simulink library "HexapodLib"  (R2014b)
settings: Solver=ode45  StartTime=0.0  StopTime=10.0  RelTol=1e-3
undefined symbols (not defined in the file): X, Y, Z
libraries: nesl_utility x95, sm_lib x85, HexapodLib x15, Contact_Forces_Lib x12
(part 2 of 3)

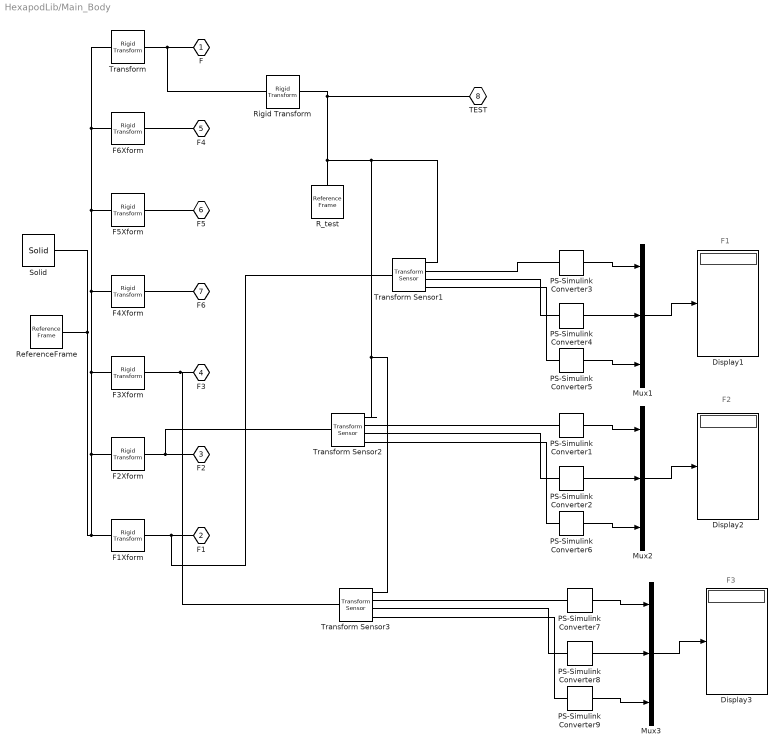
== system HexapodLib/Main_Body ==
  note: F1
  note: F2
  note: F3
  Display1 : Display
  Display2 : Display
  Display3 : Display
  F1Xform : sm_lib/Frames and Transforms/Rigid Transform  TranslationMethod=Cartesian  TranslationLengthUnit=mm  TranslationStandardAxis=+Z  TranslationStandardOffset=0  TranslationCartesianOffset=[60.910077554195617 -121.91007755419609 -2.5999999999923125]  TranslationROffset=0  TranslationROffsetUnits=m  TranslationZOffset=0  TranslationZOffsetUnits=m  TranslationThetaOffset=0  TranslationThetaOffsetUnits=deg  RotationMethod=ArbitraryAxis  RotationAngleUnits=rad  RotationStandardAxis=+Z  RotationAngle=2.3561944901923448  RotationArbitraryAxis=[-5.0947287514427085e-14 -3.4119027764489725e-14 -1]  FollAlignAxisA=+X  BaseAlignAxisA=+Y  FollAlignAxisB=+Y  BaseAlignAxisB=+Z  RotationMatrix=[1 0 0; 0 1 0; 0 0 1]  BlockFunction=simmechanics.library.frames_transforms.rigid_transform
  F2Xform : sm_lib/Frames and Transforms/Rigid Transform  TranslationMethod=Cartesian  TranslationLengthUnit=mm  TranslationStandardAxis=+Z  TranslationStandardOffset=0  TranslationCartesianOffset=[103.49999999999983 0 -2.6000000000064678]  TranslationROffset=0  TranslationROffsetUnits=m  TranslationZOffset=0  TranslationZOffsetUnits=m  TranslationThetaOffset=0  TranslationThetaOffsetUnits=deg  RotationMethod=ArbitraryAxis  RotationAngleUnits=rad  RotationStandardAxis=+Z  RotationAngle=1.5707963267948968  RotationArbitraryAxis=[-7.8558330123970482e-14 -1.5711666024794097e-14 -1]  FollAlignAxisA=+X  BaseAlignAxisA=+Y  FollAlignAxisB=+Y  BaseAlignAxisB=+Z  RotationMatrix=[1 0 0; 0 1 0; 0 0 1]  BlockFunction=simmechanics.library.frames_transforms.rigid_transform
  F3Xform : sm_lib/Frames and Transforms/Rigid Transform  TranslationMethod=Cartesian  TranslationLengthUnit=mm  TranslationStandardAxis=+Z  TranslationStandardOffset=0  TranslationCartesianOffset=[60.910077554195631 121.91007755419552 -2.6000000000152843]  TranslationROffset=0  TranslationROffsetUnits=m  TranslationZOffset=0  TranslationZOffsetUnits=m  TranslationThetaOffset=0  TranslationThetaOffsetUnits=deg  RotationMethod=ArbitraryAxis  RotationAngleUnits=rad  RotationStandardAxis=+Z  RotationAngle=0.7853981633974495  RotationArbitraryAxis=[-1.4521728366319145e-13 2.8727636334686562e-14 -1]  FollAlignAxisA=+X  BaseAlignAxisA=+Y  FollAlignAxisB=+Y  BaseAlignAxisB=+Z  RotationMatrix=[1 0 0; 0 1 0; 0 0 1]  BlockFunction=simmechanics.library.frames_transforms.rigid_transform
  F4Xform : sm_lib/Frames and Transforms/Rigid Transform  TranslationMethod=Cartesian  TranslationLengthUnit=mm  TranslationStandardAxis=+Z  TranslationStandardOffset=0  TranslationCartesianOffset=[-60.910077554195958 121.91007755419555 -2.6000000000076282]  TranslationROffset=0  TranslationROffsetUnits=m  TranslationZOffset=0  TranslationZOffsetUnits=m  TranslationThetaOffset=0  TranslationThetaOffsetUnits=deg  RotationMethod=ArbitraryAxis  RotationAngleUnits=rad  RotationStandardAxis=+Z  RotationAngle=0.78539816339744906  RotationArbitraryAxis=[-8.2370619564015128e-14 1.229976324834512e-13 1]  FollAlignAxisA=+X  BaseAlignAxisA=+Y  FollAlignAxisB=+Y  BaseAlignAxisB=+Z  RotationMatrix=[1 0 0; 0 1 0; 0 0 1]  BlockFunction=simmechanics.library.frames_transforms.rigid_transform
  F5Xform : sm_lib/Frames and Transforms/Rigid Transform  TranslationMethod=Cartesian  TranslationLengthUnit=mm  TranslationStandardAxis=+Z  TranslationStandardOffset=0  TranslationCartesianOffset=[-103.50000000000016 0 -2.5999999999934662]  TranslationROffset=0  TranslationROffsetUnits=m  TranslationZOffset=0  TranslationZOffsetUnits=m  TranslationThetaOffset=0  TranslationThetaOffsetUnits=deg  RotationMethod=ArbitraryAxis  RotationAngleUnits=rad  RotationStandardAxis=+Z  RotationAngle=1.5707963267948968  RotationArbitraryAxis=[-1.5711666024794097e-14 7.8558330123970482e-14 1]  FollAlignAxisA=+X  BaseAlignAxisA=+Y  FollAlignAxisB=+Y  BaseAlignAxisB=+Z  RotationMatrix=[1 0 0; 0 1 0; 0 0 1]  BlockFunction=simmechanics.library.frames_transforms.rigid_transform
  F6Xform : sm_lib/Frames and Transforms/Rigid Transform  TranslationMethod=Cartesian  TranslationLengthUnit=mm  TranslationStandardAxis=+Z  TranslationStandardOffset=0  TranslationCartesianOffset=[-60.910077554195937 -121.91007755419606 -2.5999999999846568]  TranslationROffset=0  TranslationROffsetUnits=m  TranslationZOffset=0  TranslationZOffsetUnits=m  TranslationThetaOffset=0  TranslationThetaOffsetUnits=deg  RotationMethod=ArbitraryAxis  RotationAngleUnits=rad  RotationStandardAxis=+Z  RotationAngle=2.3561944901923453  RotationArbitraryAxis=[1.1899376584749339e-14 6.0150968384274875e-14 1]  FollAlignAxisA=+X  BaseAlignAxisA=+Y  FollAlignAxisB=+Y  BaseAlignAxisB=+Z  RotationMatrix=[1 0 0; 0 1 0; 0 0 1]  BlockFunction=simmechanics.library.frames_transforms.rigid_transform
  Mux1 : Mux  Inputs=3
  Mux2 : Mux  Inputs=3
  Mux3 : Mux  Inputs=3
  PS-Simulink Converter{1..9} (9 alike) : nesl_utility/PS-Simulink Converter  PhysicalDomain=network_engine_domain  SubClassName=ps_output  LeftPortType=input  RightPortType=output  PseudoPeriodic=off  Frequencies=[]  Unit=mm  AffineConversion=off
  R_test : sm_lib/Frames and Transforms/Reference Frame  BlockFunction=simmechanics.library.frames_transforms.reference_frame
  ReferenceFrame : sm_lib/Frames and Transforms/Reference Frame  BlockFunction=simmechanics.library.frames_transforms.reference_frame
  Rigid Transform : sm_lib/Frames and Transforms/Rigid Transform  TranslationMethod=None  TranslationLengthUnit=m  TranslationStandardAxis=+Z  TranslationStandardOffset=0  TranslationCartesianOffset=[0 0 0]  TranslationROffset=0  TranslationROffsetUnits=m  TranslationZOffset=0  TranslationZOffsetUnits=m  TranslationThetaOffset=0  TranslationThetaOffsetUnits=deg  RotationMethod=StandardAxis  RotationAngleUnits=deg  RotationStandardAxis=+Z  RotationAngle=-180  RotationArbitraryAxis=[0 0 1]  FollAlignAxisA=+X  BaseAlignAxisA=+Y  FollAlignAxisB=+Y  BaseAlignAxisB=+Z  RotationMatrix=[1 0 0; 0 1 0; 0 0 1]  BlockFunction=simmechanics.library.frames_transforms.rigid_transform
  Solid : sm_lib/Body Elements/Solid  InertiaType=Custom  Mass=0.63100000000000001  MassUnits=kg  CenterOfMass=[2.0291292946603825 -3.6242909829433687 -16.352184508248953]  CenterOfMassUnits=mm  MomentsOfInertia=[273.36575860845227 90.65491799060328 363.95192659905558]  MomentsOfInertiaUnits=kg*mm^2  ProductsOfInertia=[0 0 0]  ProductsOfInertiaUnits=kg*mm^2  DensityBased=on  Density=1000  DensityUnits=kg/(m^3)  GraphicType=FromGeometry  MarkerShape=Sphere  MarkerSize=10  MarkerSizeUnits=m  GraphicVisPropType=SimpleVisualProperties  GraphicDiffuseColor=[0.50196078431372548 0.50196078431372548 0.50196078431372548]  GraphicSpecularColor=[0.5 0.5 0.5 1.0]  GraphicAmbientColor=[0.15 0.15 0.15 1.0]  GraphicEmissiveColor=[0.0 0.0 0.0 1.0]  GraphicShininess=75  GraphicOpacity=1  GeometryShape=FromFile  RectangleSize=[1 1]  RectangleSizeUnits=m  BrickDimensions=[1 1 1]  BrickDimensionUnits=m  CylinderRadius=1  CylinderRadiusUnits=m  CylinderLength=1  CylinderLengthUnits=m  SphereRadius=1  SphereRadiusUnits=m  EllipsoidRadii=[1 1 1]  EllipsoidRadiiUnits=m  ExtrusionCrossSection=[1 1; -1 1; -1 -1; 1 -1]  ExtrusionCrossSectionUnits=m  ExtrusionLength=1  ExtrusionLengthUnits=m  PolygonNumSides=3  PolygonOuterRadius=1  PolygonOuterRadiusUnits=m  ExtGeomFileType=STL  ExtGeomFileName=Main_body_Default_sldprt.STL  ExtGeomFileUnits=mm  RevolutionCrossSection=[1 1; 1 -1; 2 -1; 2 1]  RevolutionCrossSectionUnits=m  RevolutionExtent=Full  RevolutionAngle=180  RevolutionAngleUnits=deg  BlockFunction=simmechanics.library.body_elements.solid
  Transform : sm_lib/Frames and Transforms/Rigid Transform  TranslationMethod=Cartesian  TranslationLengthUnit=mm  TranslationStandardAxis=+Z  TranslationStandardOffset=0  TranslationCartesianOffset=[0 0 0]  TranslationROffset=0  TranslationROffsetUnits=m  TranslationZOffset=0  TranslationZOffsetUnits=m  TranslationThetaOffset=0  TranslationThetaOffsetUnits=deg  RotationMethod=ArbitraryAxis  RotationAngleUnits=rad  RotationStandardAxis=+Z  RotationAngle=0  RotationArbitraryAxis=[0 0 0]  FollAlignAxisA=+X  BaseAlignAxisA=+Y  FollAlignAxisB=+Y  BaseAlignAxisB=+Z  RotationMatrix=[1 0 0; 0 1 0; 0 0 1]  BlockFunction=simmechanics.library.frames_transforms.rigid_transform
  Transform Sensor1 : sm_lib/Frames and Transforms/Transform Sensor  MeasurementFrame=Base  SenseAngle=off  SenseAxis=off  SenseAngle1=off  SenseAngle2=off  SenseAngle3=off  SenseQ=off  SenseR=off  SenseOmegaX=off  SenseOmegaY=off  SenseOmegaZ=off  SenseOmega1=off  SenseOmega2=off  SenseOmega3=off  SenseQDot=off  SenseRDot=off  SenseAlphaX=off  SenseAlphaY=off  SenseAlphaZ=off  SenseAlpha1=off  SenseAlpha2=off  SenseAlpha3=off  SenseQDDot=off  SenseRDDot=off  SenseX=on  SenseY=on  SenseZ=on  SenseRad=off  SenseAzim=off  SenseDist=off  SenseInc=off  SenseXDot=off  SenseYDot=off  SenseZDot=off  SenseRadDot=off  SenseAzimDot=off  SenseDistDot=off  SenseIncDot=off  SenseXDDot=off  SenseYDDot=off  SenseZDDot=off  SenseRadDDot=off  SenseAzimDDot=off  SenseDistDDot=off  SenseIncDDot=off  BlockFunction=simmechanics.library.frames_transforms.transform_sensor
  Transform Sensor2 : sm_lib/Frames and Transforms/Transform Sensor  MeasurementFrame=Base  SenseAngle=off  SenseAxis=off  SenseAngle1=off  SenseAngle2=off  SenseAngle3=off  SenseQ=off  SenseR=off  SenseOmegaX=off  SenseOmegaY=off  SenseOmegaZ=off  SenseOmega1=off  SenseOmega2=off  SenseOmega3=off  SenseQDot=off  SenseRDot=off  SenseAlphaX=off  SenseAlphaY=off  SenseAlphaZ=off  SenseAlpha1=off  SenseAlpha2=off  SenseAlpha3=off  SenseQDDot=off  SenseRDDot=off  SenseX=on  SenseY=on  SenseZ=on  SenseRad=off  SenseAzim=off  SenseDist=off  SenseInc=off  SenseXDot=off  SenseYDot=off  SenseZDot=off  SenseRadDot=off  SenseAzimDot=off  SenseDistDot=off  SenseIncDot=off  SenseXDDot=off  SenseYDDot=off  SenseZDDot=off  SenseRadDDot=off  SenseAzimDDot=off  SenseDistDDot=off  SenseIncDDot=off  BlockFunction=simmechanics.library.frames_transforms.transform_sensor
  Transform Sensor3 : sm_lib/Frames and Transforms/Transform Sensor  MeasurementFrame=Base  SenseAngle=off  SenseAxis=off  SenseAngle1=off  SenseAngle2=off  SenseAngle3=off  SenseQ=off  SenseR=off  SenseOmegaX=off  SenseOmegaY=off  SenseOmegaZ=off  SenseOmega1=off  SenseOmega2=off  SenseOmega3=off  SenseQDot=off  SenseRDot=off  SenseAlphaX=off  SenseAlphaY=off  SenseAlphaZ=off  SenseAlpha1=off  SenseAlpha2=off  SenseAlpha3=off  SenseQDDot=off  SenseRDDot=off  SenseX=on  SenseY=on  SenseZ=on  SenseRad=off  SenseAzim=off  SenseDist=off  SenseInc=off  SenseXDot=off  SenseYDot=off  SenseZDot=off  SenseRadDot=off  SenseAzimDot=off  SenseDistDot=off  SenseIncDot=off  SenseXDDot=off  SenseYDDot=off  SenseZDDot=off  SenseRadDDot=off  SenseAzimDDot=off  SenseDistDDot=off  SenseIncDDot=off  BlockFunction=simmechanics.library.frames_transforms.transform_sensor
  F : PMIOPort  Port=1  Side=Left
  F1 : PMIOPort  Port=2  Side=Left
  F2 : PMIOPort  Port=3  Side=Left
  F3 : PMIOPort  Port=4  Side=Left
  F4 : PMIOPort  Port=5  Side=Right
  F5 : PMIOPort  Port=6  Side=Right
  F6 : PMIOPort  Port=7  Side=Right
  TEST : PMIOPort  Port=8  Side=Right
  wires:
  Mux1/1 -> Display1/1
  PS-Simulink Converter5/1 -> Mux1/3
  PS-Simulink Converter4/1 -> Mux1/2
  PS-Simulink Converter3/1 -> Mux1/1
  Mux2/1 -> Display2/1
  PS-Simulink Converter6/1 -> Mux2/3
  PS-Simulink Converter2/1 -> Mux2/2
  PS-Simulink Converter1/1 -> Mux2/1
  Mux3/1 -> Display3/1
  PS-Simulink Converter9/1 -> Mux3/3
  PS-Simulink Converter8/1 -> Mux3/2
  PS-Simulink Converter7/1 -> Mux3/1
  connections:
  F2Xform/LConn1 -- F6Xform/LConn1 -- Transform/LConn1 -- F5Xform/LConn1 -- F4Xform/LConn1 -- F3Xform/LConn1 -- F1Xform/LConn1 -- Solid/RConn1 -- ReferenceFrame/RConn1
  F1Xform/RConn1 -- Transform Sensor1/LConn1 -- F1/RConn1
  F2Xform/RConn1 -- Transform Sensor2/LConn1 -- F2/RConn1
  F3Xform/RConn1 -- Transform Sensor3/LConn1 -- F3/RConn1
  F4Xform/RConn1 -- F6/RConn1
  F5Xform/RConn1 -- F5/RConn1
  F6Xform/RConn1 -- F4/RConn1
  Transform/RConn1 -- Rigid Transform/LConn1 -- F/RConn1
  R_test/RConn1 -- Transform Sensor2/RConn1 -- Transform Sensor3/RConn1 -- Transform Sensor1/RConn1 -- TEST/RConn1 -- Rigid Transform/RConn1
  Transform Sensor1/RConn4 -- PS-Simulink Converter5/LConn1
  PS-Simulink Converter3/LConn1 -- Transform Sensor1/RConn2
  PS-Simulink Converter4/LConn1 -- Transform Sensor1/RConn3
  PS-Simulink Converter1/LConn1 -- Transform Sensor2/RConn2
  PS-Simulink Converter2/LConn1 -- Transform Sensor2/RConn3
  Transform Sensor2/RConn4 -- PS-Simulink Converter6/LConn1
  PS-Simulink Converter8/LConn1 -- Transform Sensor3/RConn3
  PS-Simulink Converter7/LConn1 -- Transform Sensor3/RConn2
  Transform Sensor3/RConn4 -- PS-Simulink Converter9/LConn1

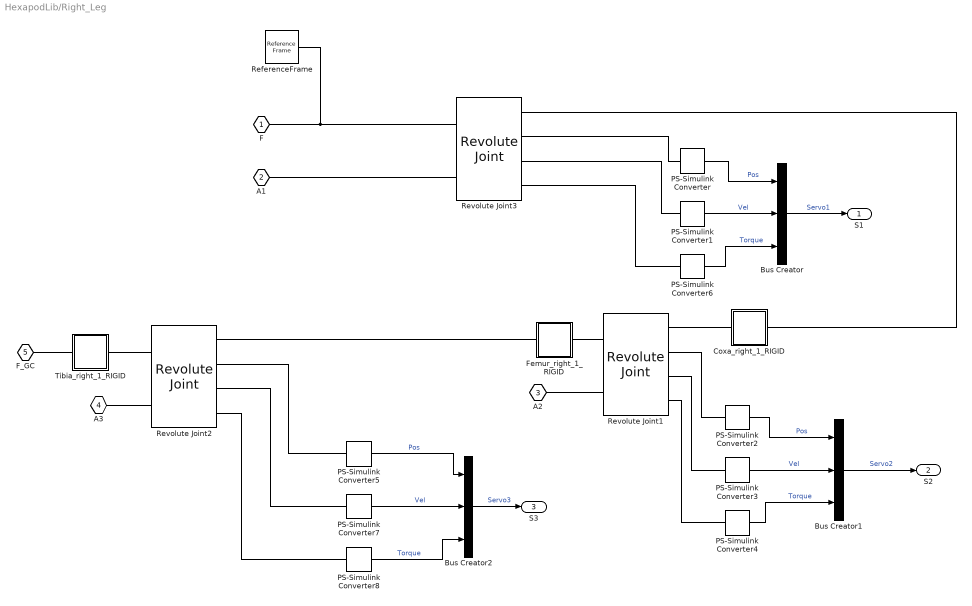
== system HexapodLib/Right_Leg ==
  Bus Creator : BusCreator  Inputs=3  OutDataTypeStr=Bus: Mes_servo
      settings: InheritFromInputs=off
  Bus Creator1 : BusCreator  Inputs=3  OutDataTypeStr=Bus: Mes_servo
      settings: InheritFromInputs=off
  Bus Creator2 : BusCreator  Inputs=3  OutDataTypeStr=Bus: Mes_servo
      settings: InheritFromInputs=off
  Coxa_right_1_RIGID : Subsystem
  Femur_right_1_RIGID : Subsystem
  PS-Simulink Converter : nesl_utility/PS-Simulink Converter  PhysicalDomain=network_engine_domain  SubClassName=ps_output  LeftPortType=input  RightPortType=output  PseudoPeriodic=off  Frequencies=[]  Unit=rad  AffineConversion=off
  PS-Simulink Converter1 : nesl_utility/PS-Simulink Converter  PhysicalDomain=network_engine_domain  SubClassName=ps_output  LeftPortType=input  RightPortType=output  PseudoPeriodic=off  Frequencies=[]  Unit=rad/s  AffineConversion=off
  PS-Simulink Converter2 : nesl_utility/PS-Simulink Converter  PhysicalDomain=network_engine_domain  SubClassName=ps_output  LeftPortType=input  RightPortType=output  PseudoPeriodic=off  Frequencies=[]  Unit=rad  AffineConversion=off
  PS-Simulink Converter3 : nesl_utility/PS-Simulink Converter  PhysicalDomain=network_engine_domain  SubClassName=ps_output  LeftPortType=input  RightPortType=output  PseudoPeriodic=off  Frequencies=[]  Unit=rad/s  AffineConversion=off
  PS-Simulink Converter4 : nesl_utility/PS-Simulink Converter  PhysicalDomain=network_engine_domain  SubClassName=ps_output  LeftPortType=input  RightPortType=output  PseudoPeriodic=off  Frequencies=[]  Unit=N*m  AffineConversion=off
  PS-Simulink Converter5 : nesl_utility/PS-Simulink Converter  PhysicalDomain=network_engine_domain  SubClassName=ps_output  LeftPortType=input  RightPortType=output  PseudoPeriodic=off  Frequencies=[]  Unit=rad  AffineConversion=off
  PS-Simulink Converter6 : nesl_utility/PS-Simulink Converter  PhysicalDomain=network_engine_domain  SubClassName=ps_output  LeftPortType=input  RightPortType=output  PseudoPeriodic=off  Frequencies=[]  Unit=N*m  AffineConversion=off
  PS-Simulink Converter7 : nesl_utility/PS-Simulink Converter  PhysicalDomain=network_engine_domain  SubClassName=ps_output  LeftPortType=input  RightPortType=output  PseudoPeriodic=off  Frequencies=[]  Unit=rad/s  AffineConversion=off
  PS-Simulink Converter8 : nesl_utility/PS-Simulink Converter  PhysicalDomain=network_engine_domain  SubClassName=ps_output  LeftPortType=input  RightPortType=output  PseudoPeriodic=off  Frequencies=[]  Unit=N*m  AffineConversion=off
  ReferenceFrame : sm_lib/Frames and Transforms/Reference Frame  BlockFunction=simmechanics.library.frames_transforms.reference_frame
  Revolute Joint1 : sm_lib/Joints/Revolute Joint  SenseConstraintForce=off  SenseConstraintForceX=off  SenseConstraintForceY=off  SenseConstraintForceZ=off  SenseConstraintTorque=off  SenseConstraintTorqueX=off  SenseConstraintTorqueY=off  SenseConstraintTorqueZ=off  SenseTotalForce=off  SenseTotalForceX=off  SenseTotalForceY=off  SenseTotalForceZ=off  SenseTotalTorque=off  SenseTotalTorqueX=off  SenseTotalTorqueY=off  SenseTotalTorqueZ=off  CompositeWrenchDir=FollowerOnBase  CompositeWrenchFrame=BaseFrame  EquilibriumPosition=0  EquilibriumPositionUnits=deg  SpringStiffness=spring_stiff  SpringStiffnessUnits=N*m/deg  DampingCoefficient=damping_coeff  DampingCoefficientUnits=N*m/(deg/s)  TorqueActuationMode=ComputedTorque  MotionActuationMode=InputMotion  SensePosition=on  SenseVelocity=on  SenseAcceleration=off  SenseTorqueForce=on  PositionTargetValue=0  PositionTargetValueUnits=deg  PositionTargetSpecify=off  PositionTargetPriority=High  VelocityTargetValue=0  VelocityTargetValueUnits=deg/s  VelocityTargetSpecify=off  VelocityTargetPriority=High  BlockFunction=simmechanics.library.joints.revolute_joint
  Revolute Joint2 : sm_lib/Joints/Revolute Joint  SenseConstraintForce=off  SenseConstraintForceX=off  SenseConstraintForceY=off  SenseConstraintForceZ=off  SenseConstraintTorque=off  SenseConstraintTorqueX=off  SenseConstraintTorqueY=off  SenseConstraintTorqueZ=off  SenseTotalForce=off  SenseTotalForceX=off  SenseTotalForceY=off  SenseTotalForceZ=off  SenseTotalTorque=off  SenseTotalTorqueX=off  SenseTotalTorqueY=off  SenseTotalTorqueZ=off  CompositeWrenchDir=FollowerOnBase  CompositeWrenchFrame=BaseFrame  EquilibriumPosition=0  EquilibriumPositionUnits=deg  SpringStiffness=spring_stiff  SpringStiffnessUnits=N*m/deg  DampingCoefficient=damping_coeff  DampingCoefficientUnits=N*m/(deg/s)  TorqueActuationMode=ComputedTorque  MotionActuationMode=InputMotion  SensePosition=on  SenseVelocity=on  SenseAcceleration=off  SenseTorqueForce=on  PositionTargetValue=0  PositionTargetValueUnits=deg  PositionTargetSpecify=off  PositionTargetPriority=High  VelocityTargetValue=0  VelocityTargetValueUnits=deg/s  VelocityTargetSpecify=off  VelocityTargetPriority=High  BlockFunction=simmechanics.library.joints.revolute_joint
  Revolute Joint3 : sm_lib/Joints/Revolute Joint  SenseConstraintForce=off  SenseConstraintForceX=off  SenseConstraintForceY=off  SenseConstraintForceZ=off  SenseConstraintTorque=off  SenseConstraintTorqueX=off  SenseConstraintTorqueY=off  SenseConstraintTorqueZ=off  SenseTotalForce=off  SenseTotalForceX=off  SenseTotalForceY=off  SenseTotalForceZ=off  SenseTotalTorque=off  SenseTotalTorqueX=off  SenseTotalTorqueY=off  SenseTotalTorqueZ=off  CompositeWrenchDir=FollowerOnBase  CompositeWrenchFrame=BaseFrame  EquilibriumPosition=0  EquilibriumPositionUnits=deg  SpringStiffness=spring_stiff  SpringStiffnessUnits=N*m/deg  DampingCoefficient=damping_coeff  DampingCoefficientUnits=N*m/(deg/s)  TorqueActuationMode=ComputedTorque  MotionActuationMode=InputMotion  SensePosition=on  SenseVelocity=on  SenseAcceleration=off  SenseTorqueForce=on  PositionTargetValue=0  PositionTargetValueUnits=deg  PositionTargetSpecify=off  PositionTargetPriority=High  VelocityTargetValue=0  VelocityTargetValueUnits=deg/s  VelocityTargetSpecify=off  VelocityTargetPriority=High  BlockFunction=simmechanics.library.joints.revolute_joint
  Tibia_right_1_RIGID : Subsystem
  F : PMIOPort  Port=1  Side=Left
  A1 : PMIOPort  Port=2  Side=Left
  A2 : PMIOPort  Port=3  Side=Left
  A3 : PMIOPort  Port=4  Side=Left
  F_GC : PMIOPort  Port=5  Side=Right
  S1 : Outport
  S2 : Outport  Port=2
  S3 : Outport  Port=3
  wires:
  Bus Creator/1 -> S1/1  "Servo1"
  PS-Simulink Converter1/1 -> Bus Creator/2  "Vel"
  PS-Simulink Converter/1 -> Bus Creator/1  "Pos"
  PS-Simulink Converter6/1 -> Bus Creator/3  "Torque"
  Bus Creator1/1 -> S2/1  "Servo2"
  PS-Simulink Converter3/1 -> Bus Creator1/2  "Vel"
  PS-Simulink Converter2/1 -> Bus Creator1/1  "Pos"
  PS-Simulink Converter4/1 -> Bus Creator1/3  "Torque"
  Bus Creator2/1 -> S3/1  "Servo3"
  PS-Simulink Converter7/1 -> Bus Creator2/2  "Vel"
  PS-Simulink Converter5/1 -> Bus Creator2/1  "Pos"
  PS-Simulink Converter8/1 -> Bus Creator2/3  "Torque"
  connections:
  Revolute Joint2/LConn2 -- A3/RConn1
  A2/RConn1 -- Revolute Joint1/LConn2
  Revolute Joint3/LConn2 -- A1/RConn1
  Revolute Joint3/RConn3 -- PS-Simulink Converter1/LConn1
  Revolute Joint3/RConn2 -- PS-Simulink Converter/LConn1
  Coxa_right_1_RIGID/LConn1 -- Revolute Joint3/RConn1
  Revolute Joint3/LConn1 -- F/RConn1 -- ReferenceFrame/RConn1
  PS-Simulink Converter6/LConn1 -- Revolute Joint3/RConn4
  Revolute Joint1/RConn3 -- PS-Simulink Converter3/LConn1
  Revolute Joint1/RConn2 -- PS-Simulink Converter2/LConn1
  Revolute Joint1/RConn4 -- PS-Simulink Converter4/LConn1
  Revolute Joint2/RConn3 -- PS-Simulink Converter7/LConn1
  Revolute Joint2/RConn2 -- PS-Simulink Converter5/LConn1
  Revolute Joint2/RConn4 -- PS-Simulink Converter8/LConn1
  F_GC/RConn1 -- Tibia_right_1_RIGID/RConn1
  Revolute Joint2/LConn1 -- Tibia_right_1_RIGID/LConn1
  Femur_right_1_RIGID/RConn1 -- Revolute Joint2/RConn1
  Revolute Joint1/LConn1 -- Femur_right_1_RIGID/LConn1
  Coxa_right_1_RIGID/RConn1 -- Revolute Joint1/RConn1

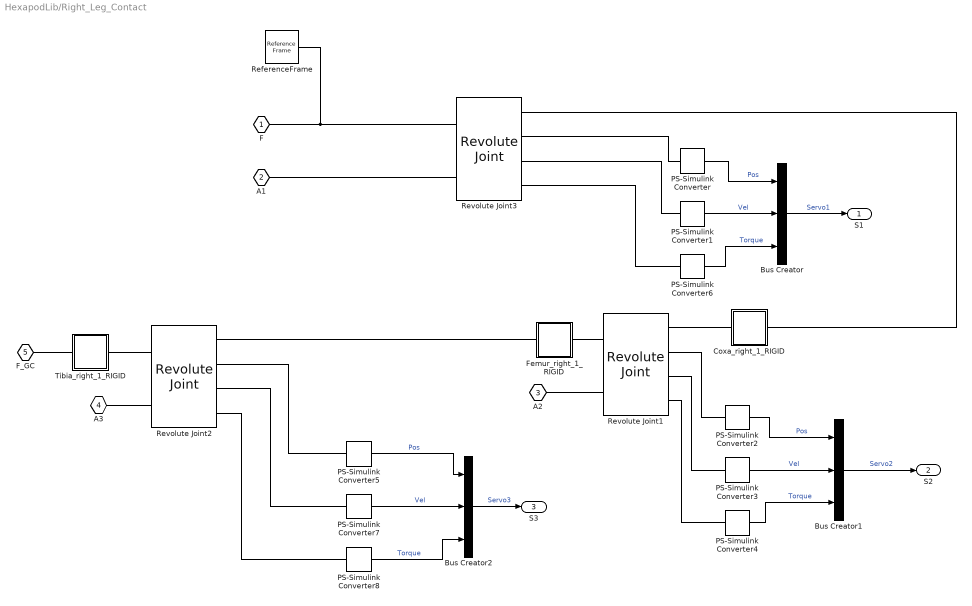
== system HexapodLib/Right_Leg_Contact ==
  Bus Creator : BusCreator  Inputs=3  OutDataTypeStr=Bus: Mes_servo
      settings: InheritFromInputs=off
  Bus Creator1 : BusCreator  Inputs=3  OutDataTypeStr=Bus: Mes_servo
      settings: InheritFromInputs=off
  Bus Creator2 : BusCreator  Inputs=3  OutDataTypeStr=Bus: Mes_servo
      settings: InheritFromInputs=off
  Coxa_right_1_RIGID : Subsystem
  Femur_right_1_RIGID : Subsystem
  PS-Simulink Converter : nesl_utility/PS-Simulink Converter  PhysicalDomain=network_engine_domain  SubClassName=ps_output  LeftPortType=input  RightPortType=output  PseudoPeriodic=off  Frequencies=[]  Unit=rad  AffineConversion=off
  PS-Simulink Converter1 : nesl_utility/PS-Simulink Converter  PhysicalDomain=network_engine_domain  SubClassName=ps_output  LeftPortType=input  RightPortType=output  PseudoPeriodic=off  Frequencies=[]  Unit=rad/s  AffineConversion=off
  PS-Simulink Converter2 : nesl_utility/PS-Simulink Converter  PhysicalDomain=network_engine_domain  SubClassName=ps_output  LeftPortType=input  RightPortType=output  PseudoPeriodic=off  Frequencies=[]  Unit=rad  AffineConversion=off
  PS-Simulink Converter3 : nesl_utility/PS-Simulink Converter  PhysicalDomain=network_engine_domain  SubClassName=ps_output  LeftPortType=input  RightPortType=output  PseudoPeriodic=off  Frequencies=[]  Unit=rad/s  AffineConversion=off
  PS-Simulink Converter4 : nesl_utility/PS-Simulink Converter  PhysicalDomain=network_engine_domain  SubClassName=ps_output  LeftPortType=input  RightPortType=output  PseudoPeriodic=off  Frequencies=[]  Unit=N*m  AffineConversion=off
  PS-Simulink Converter5 : nesl_utility/PS-Simulink Converter  PhysicalDomain=network_engine_domain  SubClassName=ps_output  LeftPortType=input  RightPortType=output  PseudoPeriodic=off  Frequencies=[]  Unit=rad  AffineConversion=off
  PS-Simulink Converter6 : nesl_utility/PS-Simulink Converter  PhysicalDomain=network_engine_domain  SubClassName=ps_output  LeftPortType=input  RightPortType=output  PseudoPeriodic=off  Frequencies=[]  Unit=N*m  AffineConversion=off
  PS-Simulink Converter7 : nesl_utility/PS-Simulink Converter  PhysicalDomain=network_engine_domain  SubClassName=ps_output  LeftPortType=input  RightPortType=output  PseudoPeriodic=off  Frequencies=[]  Unit=rad/s  AffineConversion=off
  PS-Simulink Converter8 : nesl_utility/PS-Simulink Converter  PhysicalDomain=network_engine_domain  SubClassName=ps_output  LeftPortType=input  RightPortType=output  PseudoPeriodic=off  Frequencies=[]  Unit=N*m  AffineConversion=off
  ReferenceFrame : sm_lib/Frames and Transforms/Reference Frame  BlockFunction=simmechanics.library.frames_transforms.reference_frame
  Revolute Joint1 : sm_lib/Joints/Revolute Joint  SenseConstraintForce=off  SenseConstraintForceX=off  SenseConstraintForceY=off  SenseConstraintForceZ=off  SenseConstraintTorque=off  SenseConstraintTorqueX=off  SenseConstraintTorqueY=off  SenseConstraintTorqueZ=off  SenseTotalForce=off  SenseTotalForceX=off  SenseTotalForceY=off  SenseTotalForceZ=off  SenseTotalTorque=off  SenseTotalTorqueX=off  SenseTotalTorqueY=off  SenseTotalTorqueZ=off  CompositeWrenchDir=FollowerOnBase  CompositeWrenchFrame=BaseFrame  EquilibriumPosition=0  EquilibriumPositionUnits=deg  SpringStiffness=spring_stiff  SpringStiffnessUnits=N*m/deg  DampingCoefficient=damping_coeff  DampingCoefficientUnits=N*m/(deg/s)  TorqueActuationMode=InputTorque  MotionActuationMode=ComputedMotion  SensePosition=on  SenseVelocity=on  SenseAcceleration=off  SenseTorqueForce=on  PositionTargetValue=0  PositionTargetValueUnits=deg  PositionTargetSpecify=off  PositionTargetPriority=High  VelocityTargetValue=0  VelocityTargetValueUnits=deg/s  VelocityTargetSpecify=off  VelocityTargetPriority=High  BlockFunction=simmechanics.library.joints.revolute_joint
  Revolute Joint2 : sm_lib/Joints/Revolute Joint  SenseConstraintForce=off  SenseConstraintForceX=off  SenseConstraintForceY=off  SenseConstraintForceZ=off  SenseConstraintTorque=off  SenseConstraintTorqueX=off  SenseConstraintTorqueY=off  SenseConstraintTorqueZ=off  SenseTotalForce=off  SenseTotalForceX=off  SenseTotalForceY=off  SenseTotalForceZ=off  SenseTotalTorque=off  SenseTotalTorqueX=off  SenseTotalTorqueY=off  SenseTotalTorqueZ=off  CompositeWrenchDir=FollowerOnBase  CompositeWrenchFrame=BaseFrame  EquilibriumPosition=0  EquilibriumPositionUnits=deg  SpringStiffness=spring_stiff  SpringStiffnessUnits=N*m/deg  DampingCoefficient=damping_coeff  DampingCoefficientUnits=N*m/(deg/s)  TorqueActuationMode=InputTorque  MotionActuationMode=ComputedMotion  SensePosition=on  SenseVelocity=on  SenseAcceleration=off  SenseTorqueForce=on  PositionTargetValue=0  PositionTargetValueUnits=deg  PositionTargetSpecify=off  PositionTargetPriority=High  VelocityTargetValue=0  VelocityTargetValueUnits=deg/s  VelocityTargetSpecify=off  VelocityTargetPriority=High  BlockFunction=simmechanics.library.joints.revolute_joint
  Revolute Joint3 : sm_lib/Joints/Revolute Joint  SenseConstraintForce=off  SenseConstraintForceX=off  SenseConstraintForceY=off  SenseConstraintForceZ=off  SenseConstraintTorque=off  SenseConstraintTorqueX=off  SenseConstraintTorqueY=off  SenseConstraintTorqueZ=off  SenseTotalForce=off  SenseTotalForceX=off  SenseTotalForceY=off  SenseTotalForceZ=off  SenseTotalTorque=off  SenseTotalTorqueX=off  SenseTotalTorqueY=off  SenseTotalTorqueZ=off  CompositeWrenchDir=FollowerOnBase  CompositeWrenchFrame=BaseFrame  EquilibriumPosition=0  EquilibriumPositionUnits=deg  SpringStiffness=spring_stiff  SpringStiffnessUnits=N*m/deg  DampingCoefficient=damping_coeff  DampingCoefficientUnits=N*m/(deg/s)  TorqueActuationMode=InputTorque  MotionActuationMode=ComputedMotion  SensePosition=on  SenseVelocity=on  SenseAcceleration=off  SenseTorqueForce=on  PositionTargetValue=0  PositionTargetValueUnits=deg  PositionTargetSpecify=off  PositionTargetPriority=High  VelocityTargetValue=0  VelocityTargetValueUnits=deg/s  VelocityTargetSpecify=off  VelocityTargetPriority=High  BlockFunction=simmechanics.library.joints.revolute_joint
  Tibia_right_1_RIGID : Subsystem
  F : PMIOPort  Port=1  Side=Left
  A1 : PMIOPort  Port=2  Side=Left
  A2 : PMIOPort  Port=3  Side=Left
  A3 : PMIOPort  Port=4  Side=Left
  F_GC : PMIOPort  Port=5  Side=Right
  S1 : Outport
  S2 : Outport  Port=2
  S3 : Outport  Port=3
  wires:
  Bus Creator/1 -> S1/1  "Servo1"
  PS-Simulink Converter1/1 -> Bus Creator/2  "Vel"
  PS-Simulink Converter/1 -> Bus Creator/1  "Pos"
  PS-Simulink Converter6/1 -> Bus Creator/3  "Torque"
  Bus Creator1/1 -> S2/1  "Servo2"
  PS-Simulink Converter3/1 -> Bus Creator1/2  "Vel"
  PS-Simulink Converter2/1 -> Bus Creator1/1  "Pos"
  PS-Simulink Converter4/1 -> Bus Creator1/3  "Torque"
  Bus Creator2/1 -> S3/1  "Servo3"
  PS-Simulink Converter7/1 -> Bus Creator2/2  "Vel"
  PS-Simulink Converter5/1 -> Bus Creator2/1  "Pos"
  PS-Simulink Converter8/1 -> Bus Creator2/3  "Torque"
  connections:
  Revolute Joint2/LConn2 -- A3/RConn1
  A2/RConn1 -- Revolute Joint1/LConn2
  Revolute Joint3/LConn2 -- A1/RConn1
  Revolute Joint3/RConn3 -- PS-Simulink Converter1/LConn1
  Revolute Joint3/RConn2 -- PS-Simulink Converter/LConn1
  Coxa_right_1_RIGID/LConn1 -- Revolute Joint3/RConn1
  Revolute Joint3/LConn1 -- F/RConn1 -- ReferenceFrame/RConn1
  PS-Simulink Converter6/LConn1 -- Revolute Joint3/RConn4
  Revolute Joint1/RConn3 -- PS-Simulink Converter3/LConn1
  Revolute Joint1/RConn2 -- PS-Simulink Converter2/LConn1
  Revolute Joint1/RConn4 -- PS-Simulink Converter4/LConn1
  Revolute Joint2/RConn3 -- PS-Simulink Converter7/LConn1
  Revolute Joint2/RConn2 -- PS-Simulink Converter5/LConn1
  Revolute Joint2/RConn4 -- PS-Simulink Converter8/LConn1
  F_GC/RConn1 -- Tibia_right_1_RIGID/RConn1
  Revolute Joint2/LConn1 -- Tibia_right_1_RIGID/LConn1
  Femur_right_1_RIGID/RConn1 -- Revolute Joint2/RConn1
  Revolute Joint1/LConn1 -- Femur_right_1_RIGID/LConn1
  Coxa_right_1_RIGID/RConn1 -- Revolute Joint1/RConn1

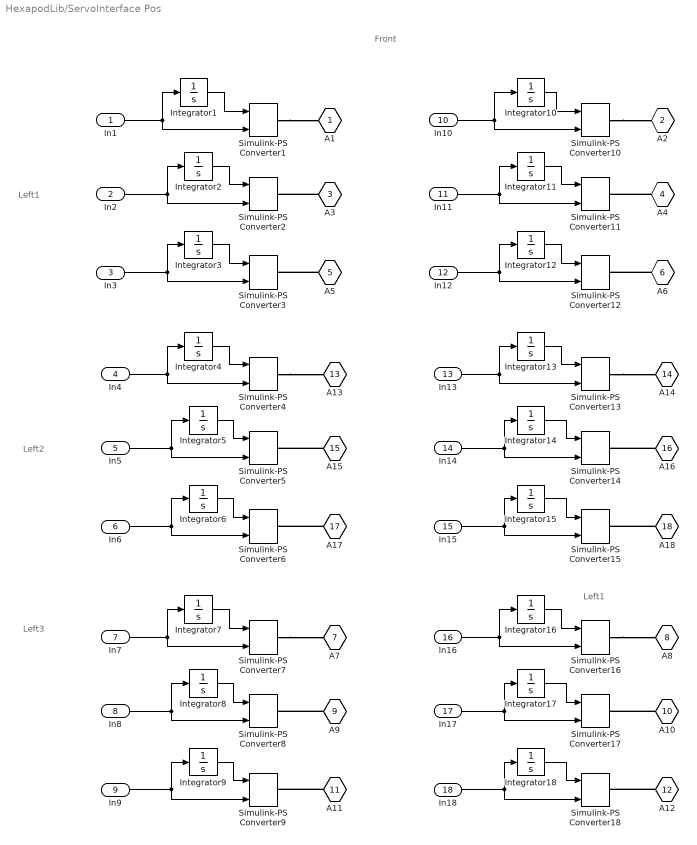
== system HexapodLib/ServoInterface Pos ==
  note: Front
  note: Left1
  note: Left2
  note: Left1
  note: Left3
  In1 : Inport
  In2 : Inport  Port=2
  In3 : Inport  Port=3
  In4 : Inport  Port=4
  In5 : Inport  Port=5
  In6 : Inport  Port=6
  In7 : Inport  Port=7
  In8 : Inport  Port=8
  In9 : Inport  Port=9
  In10 : Inport  Port=10
  In11 : Inport  Port=11
  In12 : Inport  Port=12
  In13 : Inport  Port=13
  In14 : Inport  Port=14
  In15 : Inport  Port=15
  In16 : Inport  Port=16
  In17 : Inport  Port=17
  In18 : Inport  Port=18
  Integrator{1..18} (18 alike) : Integrator
  Simulink-PS Converter{1..18} (18 alike) : nesl_utility/Simulink-PS Converter  PhysicalDomain=network_engine_domain  SubClassName=ps_input  LeftPortType=input  RightPortType=output  PseudoPeriodic=off  Frequencies=[]  NoiseDistribution=none  NoiseParameters=[]  Unit=deg  AffineConversion=off  InputFiltering=derivs  SimscapeFilterOrder=1  InputFilterTimeConstant=0.001  UdotUserProvided=1
  A1 : PMIOPort  Port=1  Side=Right
  A2 : PMIOPort  Port=2  Side=Right
  A3 : PMIOPort  Port=3  Side=Right
  A4 : PMIOPort  Port=4  Side=Right
  A5 : PMIOPort  Port=5  Side=Right
  A6 : PMIOPort  Port=6  Side=Right
  A7 : PMIOPort  Port=7  Side=Right
  A8 : PMIOPort  Port=8  Side=Right
  A9 : PMIOPort  Port=9  Side=Right
  A10 : PMIOPort  Port=10  Side=Right
  A11 : PMIOPort  Port=11  Side=Right
  A12 : PMIOPort  Port=12  Side=Right
  A13 : PMIOPort  Port=13  Side=Right
  A14 : PMIOPort  Port=14  Side=Right
  A15 : PMIOPort  Port=15  Side=Right
  A16 : PMIOPort  Port=16  Side=Right
  A17 : PMIOPort  Port=17  Side=Right
  A18 : PMIOPort  Port=18  Side=Right
  wires:
  Integrator1/1 -> Simulink-PS Converter1/1
  In1/1 -> Integrator1/1, Simulink-PS Converter1/2
  Integrator2/1 -> Simulink-PS Converter2/1
  In2/1 -> Integrator2/1, Simulink-PS Converter2/2
  Integrator3/1 -> Simulink-PS Converter3/1
  In3/1 -> Integrator3/1, Simulink-PS Converter3/2
  Integrator4/1 -> Simulink-PS Converter4/1
  In4/1 -> Integrator4/1, Simulink-PS Converter4/2
  Integrator5/1 -> Simulink-PS Converter5/1
  In5/1 -> Integrator5/1, Simulink-PS Converter5/2
  Integrator6/1 -> Simulink-PS Converter6/1
  In6/1 -> Integrator6/1, Simulink-PS Converter6/2
  Integrator7/1 -> Simulink-PS Converter7/1
  In7/1 -> Integrator7/1, Simulink-PS Converter7/2
  Integrator8/1 -> Simulink-PS Converter8/1
  In8/1 -> Integrator8/1, Simulink-PS Converter8/2
  Integrator9/1 -> Simulink-PS Converter9/1
  In9/1 -> Integrator9/1, Simulink-PS Converter9/2
  Integrator10/1 -> Simulink-PS Converter10/1
  In10/1 -> Integrator10/1, Simulink-PS Converter10/2
  Integrator11/1 -> Simulink-PS Converter11/1
  In11/1 -> Integrator11/1, Simulink-PS Converter11/2
  Integrator12/1 -> Simulink-PS Converter12/1
  In12/1 -> Integrator12/1, Simulink-PS Converter12/2
  Integrator13/1 -> Simulink-PS Converter13/1
  In13/1 -> Integrator13/1, Simulink-PS Converter13/2
  Integrator14/1 -> Simulink-PS Converter14/1
  In14/1 -> Integrator14/1, Simulink-PS Converter14/2
  Integrator15/1 -> Simulink-PS Converter15/1
  In15/1 -> Integrator15/1, Simulink-PS Converter15/2
  Integrator16/1 -> Simulink-PS Converter16/1
  In16/1 -> Integrator16/1, Simulink-PS Converter16/2
  Integrator17/1 -> Simulink-PS Converter17/1
  In17/1 -> Integrator17/1, Simulink-PS Converter17/2
  Integrator18/1 -> Simulink-PS Converter18/1
  In18/1 -> Integrator18/1, Simulink-PS Converter18/2
  connections:
  Simulink-PS Converter1/RConn1 -- A1/RConn1
  A3/RConn1 -- Simulink-PS Converter2/RConn1
  A5/RConn1 -- Simulink-PS Converter3/RConn1
  Simulink-PS Converter4/RConn1 -- A13/RConn1
  A15/RConn1 -- Simulink-PS Converter5/RConn1
  A17/RConn1 -- Simulink-PS Converter6/RConn1
  Simulink-PS Converter7/RConn1 -- A7/RConn1
  A9/RConn1 -- Simulink-PS Converter8/RConn1
  A11/RConn1 -- Simulink-PS Converter9/RConn1
  A6/RConn1 -- Simulink-PS Converter12/RConn1
  Simulink-PS Converter13/RConn1 -- A14/RConn1
  A10/RConn1 -- Simulink-PS Converter17/RConn1
  Simulink-PS Converter16/RConn1 -- A8/RConn1
  A16/RConn1 -- Simulink-PS Converter14/RConn1
  A4/RConn1 -- Simulink-PS Converter11/RConn1
  A18/RConn1 -- Simulink-PS Converter15/RConn1
  Simulink-PS Converter10/RConn1 -- A2/RConn1
  A12/RConn1 -- Simulink-PS Converter18/RConn1

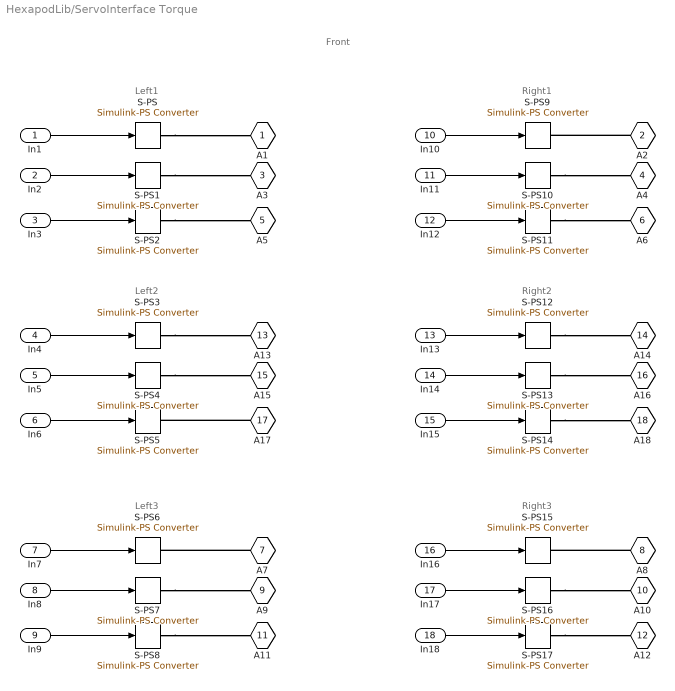
== system HexapodLib/ServoInterface Torque ==
  note: Front
  note: Left1
  note: Left2
  note: Left3
  note: Right1
  note: Right2
  note: Right3
  In1 : Inport
  In2 : Inport  Port=2
  In3 : Inport  Port=3
  In4 : Inport  Port=4
  In5 : Inport  Port=5
  In6 : Inport  Port=6
  In7 : Inport  Port=7
  In8 : Inport  Port=8
  In9 : Inport  Port=9
  In10 : Inport  Port=10
  In11 : Inport  Port=11
  In12 : Inport  Port=12
  In13 : Inport  Port=13
  In14 : Inport  Port=14
  In15 : Inport  Port=15
  In16 : Inport  Port=16
  In17 : Inport  Port=17
  In18 : Inport  Port=18
  S-PS{,1..17} (18 alike) : nesl_utility/Simulink-PS Converter  PhysicalDomain=network_engine_domain  SubClassName=ps_input  LeftPortType=input  RightPortType=output  PseudoPeriodic=off  Frequencies=[]  NoiseDistribution=none  NoiseParameters=[]  Unit=N*m  AffineConversion=off  InputFiltering=off  SimscapeFilterOrder=1  InputFilterTimeConstant=0.001  UdotUserProvided=1
  A1 : PMIOPort  Port=1  Side=Right
  A2 : PMIOPort  Port=2  Side=Right
  A3 : PMIOPort  Port=3  Side=Right
  A4 : PMIOPort  Port=4  Side=Right
  A5 : PMIOPort  Port=5  Side=Right
  A6 : PMIOPort  Port=6  Side=Right
  A7 : PMIOPort  Port=7  Side=Right
  A8 : PMIOPort  Port=8  Side=Right
  A9 : PMIOPort  Port=9  Side=Right
  A10 : PMIOPort  Port=10  Side=Right
  A11 : PMIOPort  Port=11  Side=Right
  A12 : PMIOPort  Port=12  Side=Right
  A13 : PMIOPort  Port=13  Side=Right
  A14 : PMIOPort  Port=14  Side=Right
  A15 : PMIOPort  Port=15  Side=Right
  A16 : PMIOPort  Port=16  Side=Right
  A17 : PMIOPort  Port=17  Side=Right
  A18 : PMIOPort  Port=18  Side=Right
  wires:
  In1/1 -> S-PS/1
  In2/1 -> S-PS1/1
  In3/1 -> S-PS2/1
  In4/1 -> S-PS3/1
  In5/1 -> S-PS4/1
  In6/1 -> S-PS5/1
  In7/1 -> S-PS6/1
  In8/1 -> S-PS7/1
  In9/1 -> S-PS8/1
  In10/1 -> S-PS9/1
  In11/1 -> S-PS10/1
  In12/1 -> S-PS11/1
  In13/1 -> S-PS12/1
  In14/1 -> S-PS13/1
  In15/1 -> S-PS14/1
  In16/1 -> S-PS15/1
  In17/1 -> S-PS16/1
  In18/1 -> S-PS17/1
  connections:
  S-PS/RConn1 -- A1/RConn1
  S-PS1/RConn1 -- A3/RConn1
  S-PS2/RConn1 -- A5/RConn1
  A2/RConn1 -- S-PS9/RConn1
  S-PS10/RConn1 -- A4/RConn1
  S-PS11/RConn1 -- A6/RConn1
  A17/RConn1 -- S-PS5/RConn1
  S-PS4/RConn1 -- A15/RConn1
  S-PS3/RConn1 -- A13/RConn1
  S-PS12/RConn1 -- A14/RConn1
  S-PS13/RConn1 -- A16/RConn1
  S-PS14/RConn1 -- A18/RConn1
  A7/RConn1 -- S-PS6/RConn1
  S-PS7/RConn1 -- A9/RConn1
  S-PS8/RConn1 -- A11/RConn1
  A8/RConn1 -- S-PS15/RConn1
  S-PS16/RConn1 -- A10/RConn1
  S-PS17/RConn1 -- A12/RConn1

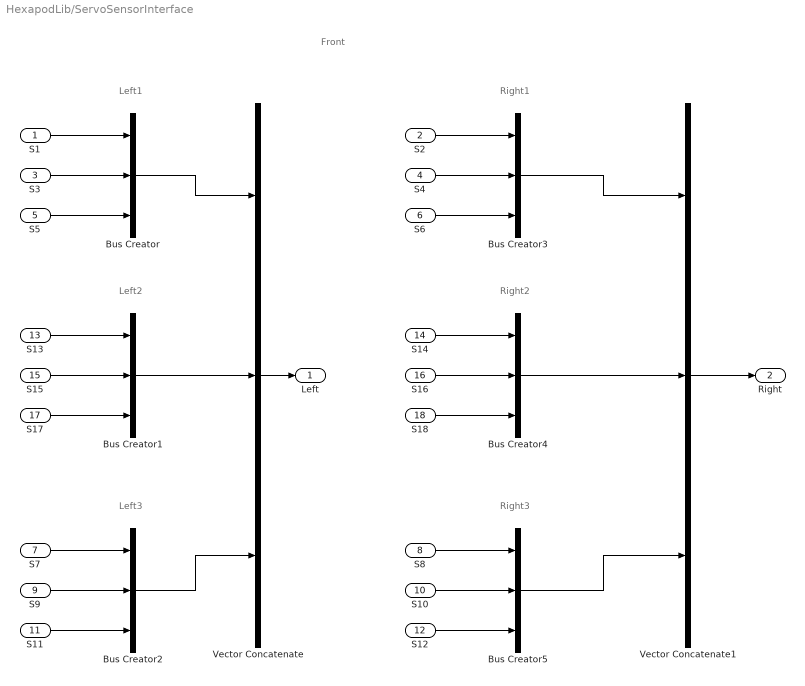
== system HexapodLib/ServoSensorInterface ==
  note: Front
  note: Left1
  note: Left2
  note: Left3
  note: Right1
  note: Right2
  note: Right3
  S1 : Inport
  S2 : Inport  Port=2
  S3 : Inport  Port=3
  S4 : Inport  Port=4
  S5 : Inport  Port=5
  S6 : Inport  Port=6
  S7 : Inport  Port=7
  S8 : Inport  Port=8
  S9 : Inport  Port=9
  S10 : Inport  Port=10
  S11 : Inport  Port=11
  S12 : Inport  Port=12
  S13 : Inport  Port=13
  S14 : Inport  Port=14
  S15 : Inport  Port=15
  S16 : Inport  Port=16
  S17 : Inport  Port=17
  S18 : Inport  Port=18
  Bus Creator{,1..5} (6 alike) : BusCreator  Inputs=3  OutDataTypeStr=Bus: Leg_mes  NonVirtualBus=on
  Vector Concatenate : Concatenate  NumInputs=3  ConcatenateDimension=2
  Vector Concatenate1 : Concatenate  NumInputs=3  ConcatenateDimension=2
  Left : Outport
  Right : Outport  Port=2
  wires:
  Bus Creator1/1 -> Vector Concatenate/2
  Bus Creator2/1 -> Vector Concatenate/3
  Bus Creator3/1 -> Vector Concatenate1/1
  Bus Creator5/1 -> Vector Concatenate1/3
  S2/1 -> Bus Creator3/1
  S4/1 -> Bus Creator3/2
  S6/1 -> Bus Creator3/3
  S14/1 -> Bus Creator4/1
  S16/1 -> Bus Creator4/2
  S18/1 -> Bus Creator4/3
  S8/1 -> Bus Creator5/1
  S10/1 -> Bus Creator5/2
  S12/1 -> Bus Creator5/3
  S1/1 -> Bus Creator/1
  S3/1 -> Bus Creator/2
  S5/1 -> Bus Creator/3
  S13/1 -> Bus Creator1/1
  S15/1 -> Bus Creator1/2
  S17/1 -> Bus Creator1/3
  S7/1 -> Bus Creator2/1
  S9/1 -> Bus Creator2/2
  S11/1 -> Bus Creator2/3
  Bus Creator/1 -> Vector Concatenate/1
  Vector Concatenate/1 -> Left/1
  Bus Creator4/1 -> Vector Concatenate1/2
  Vector Concatenate1/1 -> Right/1

== system HexapodLib/Left_Leg/Coxa_left_3_RIGID1 ==
  FXform : sm_lib/Frames and Transforms/Rigid Transform  TranslationMethod=Cartesian  TranslationLengthUnit=mm  TranslationStandardAxis=+Z  TranslationStandardOffset=0  TranslationCartesianOffset=[14.299679915594941 52.999999999368015 -14.29967991559503]  TranslationROffset=0  TranslationROffsetUnits=m  TranslationZOffset=0  TranslationZOffsetUnits=m  TranslationThetaOffset=0  TranslationThetaOffsetUnits=deg  RotationMethod=ArbitraryAxis  RotationAngleUnits=rad  RotationStandardAxis=+Z  RotationAngle=3.1415926535897931  RotationArbitraryAxis=[-0.70710678118654746 9.6907767202698026e-18 -0.70710678118654757]  FollAlignAxisA=+X  BaseAlignAxisA=+Y  FollAlignAxisB=+Y  BaseAlignAxisB=+Z  RotationMatrix=[1 0 0; 0 1 0; 0 0 1]  BlockFunction=simmechanics.library.frames_transforms.rigid_transform
  ReferenceFrame : sm_lib/Frames and Transforms/Reference Frame  BlockFunction=simmechanics.library.frames_transforms.reference_frame
  Solid : sm_lib/Body Elements/Solid  InertiaType=Custom  Mass=0.023996850766747905  MassUnits=kg  CenterOfMass=[0.93906891947679294 26.499999999684 -13.360610996118144]  CenterOfMassUnits=mm  MomentsOfInertia=[1.9924370956103432 0.50396195080190453 1.9924370956103437]  MomentsOfInertiaUnits=kg*mm^2  ProductsOfInertia=[0.59797945054951396 0.21411025390203908 -0.59797945054951407]  ProductsOfInertiaUnits=kg*mm^2  DensityBased=on  Density=1000  DensityUnits=kg/(m^3)  GraphicType=FromGeometry  MarkerShape=Sphere  MarkerSize=10  MarkerSizeUnits=m  GraphicVisPropType=SimpleVisualProperties  GraphicDiffuseColor=[0.90980392156862744 0.44313725490196076 0.031372549019607843]  GraphicSpecularColor=[0.5 0.5 0.5 1.0]  GraphicAmbientColor=[0.15 0.15 0.15 1.0]  GraphicEmissiveColor=[0.0 0.0 0.0 1.0]  GraphicShininess=75  GraphicOpacity=1  GeometryShape=FromFile  RectangleSize=[1 1]  RectangleSizeUnits=m  BrickDimensions=[1 1 1]  BrickDimensionUnits=m  CylinderRadius=1  CylinderRadiusUnits=m  CylinderLength=1  CylinderLengthUnits=m  SphereRadius=1  SphereRadiusUnits=m  EllipsoidRadii=[1 1 1]  EllipsoidRadiiUnits=m  ExtrusionCrossSection=[1 1; -1 1; -1 -1; 1 -1]  ExtrusionCrossSectionUnits=m  ExtrusionLength=1  ExtrusionLengthUnits=m  PolygonNumSides=3  PolygonOuterRadius=1  PolygonOuterRadiusUnits=m  ExtGeomFileType=STL  ExtGeomFileName=Coxa_left_Default_sldprt.STL  ExtGeomFileUnits=mm  RevolutionCrossSection=[1 1; 1 -1; 2 -1; 2 1]  RevolutionCrossSectionUnits=m  RevolutionExtent=Full  RevolutionAngle=180  RevolutionAngleUnits=deg  BlockFunction=simmechanics.library.body_elements.solid
  F1 : PMIOPort  Port=1  Side=Left
  F : PMIOPort  Port=2  Side=Right
  connections:
  FXform/LConn1 -- ReferenceFrame/RConn1 -- Solid/RConn1 -- F1/RConn1
  FXform/RConn1 -- F/RConn1

== system HexapodLib/Left_Leg/Femur_left_3_RIGID1 ==
  FXform : sm_lib/Frames and Transforms/Rigid Transform  TranslationMethod=Cartesian  TranslationLengthUnit=mm  TranslationStandardAxis=+Z  TranslationStandardOffset=0  TranslationCartesianOffset=[-14.542587190940528 -64.500041047761613 0.90030378794519206]  TranslationROffset=0  TranslationROffsetUnits=m  TranslationZOffset=0  TranslationZOffsetUnits=m  TranslationThetaOffset=0  TranslationThetaOffsetUnits=deg  RotationMethod=None  RotationAngleUnits=deg  RotationStandardAxis=+Z  RotationAngle=0.0  RotationArbitraryAxis=[0 0 1]  FollAlignAxisA=+X  BaseAlignAxisA=+Y  FollAlignAxisB=+Y  BaseAlignAxisB=+Z  RotationMatrix=[1 0 0; 0 1 0; 0 0 1]  BlockFunction=simmechanics.library.frames_transforms.rigid_transform
  ReferenceFrame : sm_lib/Frames and Transforms/Reference Frame  BlockFunction=simmechanics.library.frames_transforms.reference_frame
  Solid : sm_lib/Body Elements/Solid  InertiaType=Custom  Mass=0.072457341696858593  MassUnits=kg  CenterOfMass=[-0.44803713076721907 -21.992678596043948 -12.681987437137396]  CenterOfMassUnits=mm  MomentsOfInertia=[0.037680215126497711 0.037870673191187171 0.070577312448876009]  MomentsOfInertiaUnits=kg*mm^2  ProductsOfInertia=[-2.3976312573726778e-07 -2.4153863023073146e-08 -5.6424127328969219e-07]  ProductsOfInertiaUnits=kg*mm^2  DensityBased=on  Density=1000  DensityUnits=kg/(m^3)  GraphicType=FromGeometry  MarkerShape=Sphere  MarkerSize=10  MarkerSizeUnits=m  GraphicVisPropType=SimpleVisualProperties  GraphicDiffuseColor=[0 1 0]  GraphicSpecularColor=[0.5 0.5 0.5 1.0]  GraphicAmbientColor=[0.15 0.15 0.15 1.0]  GraphicEmissiveColor=[0.0 0.0 0.0 1.0]  GraphicShininess=75  GraphicOpacity=1  GeometryShape=FromFile  RectangleSize=[1 1]  RectangleSizeUnits=m  BrickDimensions=[1 1 1]  BrickDimensionUnits=m  CylinderRadius=1  CylinderRadiusUnits=m  CylinderLength=1  CylinderLengthUnits=m  SphereRadius=1  SphereRadiusUnits=m  EllipsoidRadii=[1 1 1]  EllipsoidRadiiUnits=m  ExtrusionCrossSection=[1 1; -1 1; -1 -1; 1 -1]  ExtrusionCrossSectionUnits=m  ExtrusionLength=1  ExtrusionLengthUnits=m  PolygonNumSides=3  PolygonOuterRadius=1  PolygonOuterRadiusUnits=m  ExtGeomFileType=STL  ExtGeomFileName=Femur_left_Default_sldprt.STL  ExtGeomFileUnits=mm  RevolutionCrossSection=[1 1; 1 -1; 2 -1; 2 1]  RevolutionCrossSectionUnits=m  RevolutionExtent=Full  RevolutionAngle=180  RevolutionAngleUnits=deg  BlockFunction=simmechanics.library.body_elements.solid
  F1 : PMIOPort  Port=1  Side=Left
  F : PMIOPort  Port=2  Side=Right
  connections:
  FXform/LConn1 -- ReferenceFrame/RConn1 -- Solid/RConn1 -- F1/RConn1
  FXform/RConn1 -- F/RConn1

== system HexapodLib/Left_Leg/Tibia_left_3_RIGID ==
  F_GCXform : sm_lib/Frames and Transforms/Rigid Transform  TranslationMethod=Cartesian  TranslationLengthUnit=mm  TranslationStandardAxis=+Z  TranslationStandardOffset=0  TranslationCartesianOffset=[-96.256056895188493 -92.416305539220545 -13.399999999999935]  TranslationROffset=0  TranslationROffsetUnits=m  TranslationZOffset=0  TranslationZOffsetUnits=m  TranslationThetaOffset=0  TranslationThetaOffsetUnits=deg  RotationMethod=ArbitraryAxis  RotationAngleUnits=rad  RotationStandardAxis=+Z  RotationAngle=0.54874368836751786  RotationArbitraryAxis=[7.0306914223032609e-16 2.4978424328474419e-15 1]  FollAlignAxisA=+X  BaseAlignAxisA=+Y  FollAlignAxisB=+Y  BaseAlignAxisB=+Z  RotationMatrix=[1 0 0; 0 1 0; 0 0 1]  BlockFunction=simmechanics.library.frames_transforms.rigid_transform
  ReferenceFrame : sm_lib/Frames and Transforms/Reference Frame  BlockFunction=simmechanics.library.frames_transforms.reference_frame
  Solid : sm_lib/Body Elements/Solid  InertiaType=Custom  Mass=0.099231623343163863  MassUnits=kg  CenterOfMass=[-20.505850411396018 -36.538235157551448 -13.103099392882958]  CenterOfMassUnits=mm  MomentsOfInertia=[0.0019304534059169495 0.0015883684234285318 0.0013841810987472742]  MomentsOfInertiaUnits=kg*mm^2  ProductsOfInertia=[0 0 0.00033397886302644037]  ProductsOfInertiaUnits=kg*mm^2  DensityBased=on  Density=1000  DensityUnits=kg/(m^3)  GraphicType=FromGeometry  MarkerShape=Sphere  MarkerSize=10  MarkerSizeUnits=m  GraphicVisPropType=SimpleVisualProperties  GraphicDiffuseColor=[0 0 1]  GraphicSpecularColor=[0.5 0.5 0.5 1.0]  GraphicAmbientColor=[0.15 0.15 0.15 1.0]  GraphicEmissiveColor=[0.0 0.0 0.0 1.0]  GraphicShininess=75  GraphicOpacity=1  GeometryShape=FromFile  RectangleSize=[1 1]  RectangleSizeUnits=m  BrickDimensions=[1 1 1]  BrickDimensionUnits=m  CylinderRadius=1  CylinderRadiusUnits=m  CylinderLength=1  CylinderLengthUnits=m  SphereRadius=1  SphereRadiusUnits=m  EllipsoidRadii=[1 1 1]  EllipsoidRadiiUnits=m  ExtrusionCrossSection=[1 1; -1 1; -1 -1; 1 -1]  ExtrusionCrossSectionUnits=m  ExtrusionLength=1  ExtrusionLengthUnits=m  PolygonNumSides=3  PolygonOuterRadius=1  PolygonOuterRadiusUnits=m  ExtGeomFileType=STL  ExtGeomFileName=Tibia_left_Default_sldprt.STL  ExtGeomFileUnits=mm  RevolutionCrossSection=[1 1; 1 -1; 2 -1; 2 1]  RevolutionCrossSectionUnits=m  RevolutionExtent=Full  RevolutionAngle=180  RevolutionAngleUnits=deg  BlockFunction=simmechanics.library.body_elements.solid
  F : PMIOPort  Port=1  Side=Left
  F_GC : PMIOPort  Port=2  Side=Right
  connections:
  F_GCXform/LConn1 -- ReferenceFrame/RConn1 -- Solid/RConn1 -- F/RConn1
  F_GCXform/RConn1 -- F_GC/RConn1

== system HexapodLib/Left_Leg_Contact/Coxa_left_3_RIGID1 ==
  FXform : sm_lib/Frames and Transforms/Rigid Transform  TranslationMethod=Cartesian  TranslationLengthUnit=mm  TranslationStandardAxis=+Z  TranslationStandardOffset=0  TranslationCartesianOffset=[14.299679915594941 52.999999999368015 -14.29967991559503]  TranslationROffset=0  TranslationROffsetUnits=m  TranslationZOffset=0  TranslationZOffsetUnits=m  TranslationThetaOffset=0  TranslationThetaOffsetUnits=deg  RotationMethod=ArbitraryAxis  RotationAngleUnits=rad  RotationStandardAxis=+Z  RotationAngle=3.1415926535897931  RotationArbitraryAxis=[-0.70710678118654746 9.6907767202698026e-18 -0.70710678118654757]  FollAlignAxisA=+X  BaseAlignAxisA=+Y  FollAlignAxisB=+Y  BaseAlignAxisB=+Z  RotationMatrix=[1 0 0; 0 1 0; 0 0 1]  BlockFunction=simmechanics.library.frames_transforms.rigid_transform
  ReferenceFrame : sm_lib/Frames and Transforms/Reference Frame  BlockFunction=simmechanics.library.frames_transforms.reference_frame
  Solid : sm_lib/Body Elements/Solid  InertiaType=Custom  Mass=0.023996850766747905  MassUnits=kg  CenterOfMass=[0.93906891947679294 26.499999999684 -13.360610996118144]  CenterOfMassUnits=mm  MomentsOfInertia=[1.9924370956103432 0.50396195080190453 1.9924370956103437]  MomentsOfInertiaUnits=kg*mm^2  ProductsOfInertia=[0.59797945054951396 0.21411025390203908 -0.59797945054951407]  ProductsOfInertiaUnits=kg*mm^2  DensityBased=on  Density=1000  DensityUnits=kg/(m^3)  GraphicType=FromGeometry  MarkerShape=Sphere  MarkerSize=10  MarkerSizeUnits=m  GraphicVisPropType=SimpleVisualProperties  GraphicDiffuseColor=[0.90980392156862744 0.44313725490196076 0.031372549019607843]  GraphicSpecularColor=[0.5 0.5 0.5 1.0]  GraphicAmbientColor=[0.15 0.15 0.15 1.0]  GraphicEmissiveColor=[0.0 0.0 0.0 1.0]  GraphicShininess=75  GraphicOpacity=1  GeometryShape=FromFile  RectangleSize=[1 1]  RectangleSizeUnits=m  BrickDimensions=[1 1 1]  BrickDimensionUnits=m  CylinderRadius=1  CylinderRadiusUnits=m  CylinderLength=1  CylinderLengthUnits=m  SphereRadius=1  SphereRadiusUnits=m  EllipsoidRadii=[1 1 1]  EllipsoidRadiiUnits=m  ExtrusionCrossSection=[1 1; -1 1; -1 -1; 1 -1]  ExtrusionCrossSectionUnits=m  ExtrusionLength=1  ExtrusionLengthUnits=m  PolygonNumSides=3  PolygonOuterRadius=1  PolygonOuterRadiusUnits=m  ExtGeomFileType=STL  ExtGeomFileName=Coxa_left_Default_sldprt.STL  ExtGeomFileUnits=mm  RevolutionCrossSection=[1 1; 1 -1; 2 -1; 2 1]  RevolutionCrossSectionUnits=m  RevolutionExtent=Full  RevolutionAngle=180  RevolutionAngleUnits=deg  BlockFunction=simmechanics.library.body_elements.solid
  F1 : PMIOPort  Port=1  Side=Left
  F : PMIOPort  Port=2  Side=Right
  connections:
  FXform/LConn1 -- ReferenceFrame/RConn1 -- Solid/RConn1 -- F1/RConn1
  FXform/RConn1 -- F/RConn1
